simulink model "A_Novel_Converter_Topology_for_Stand_Alone"  (Simulink 7.3)
settings: Solver=ode45  StartTime=0.0  StopTime=0.7  MaxStep=1e-6  RelTol=1e-3
libraries: powerlib x20
settings Model: Creator=KARTHIK  LastModifiedBy=91889
settings DebuggingCC: FcnCallInpInsideContextMsg=Enable All  StrictBusMsg=ErrorLevel1
settings GRTTargetCC: CombineOutputUpdateFcns=on

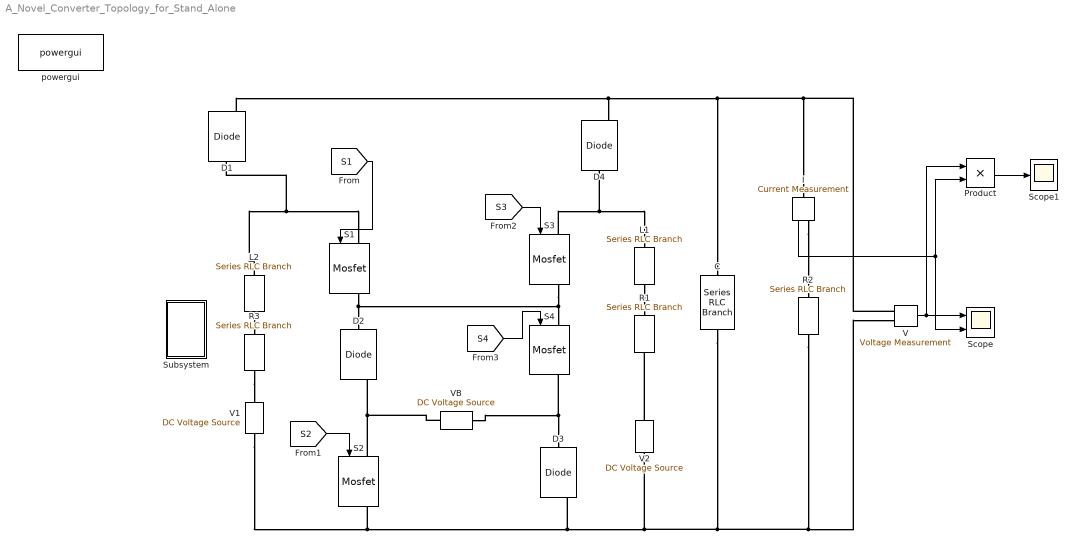
== system A_Novel_Converter_Topology_for_Stand_Alone ==
  C : powerlib/Elements/Series RLC Branch  DialogController=POWERSYS.PowerSysDialog  PhysicalDomain=powersysdomain  SubClassName=unknown  LeftPortType=p1  RightPortType=p1  LConnTagsString=__new0  RConnTagsString=__new0  BranchType=C  Resistance=1  Inductance=1e-3  SetiL0=off  InitialCurrent=0  Capacitance=200e-6  Setx0=off  InitialVoltage=0  Measurements=None
  D{1..4} (4 alike) : powerlib/Power Electronics/Diode  DialogController=POWERSYS.PowerSysDialog  SystemSampleTime=-1  Ron=0.001  Lon=0  Vf=0.8  IC=0  UseSnubber=off  Rs=500  Cs=250e-9  Measurements=on
  I : powerlib/Measurements/Current Measurement  DialogController=POWERSYS.PowerSysDialog  SystemSampleTime=-1  PhasorSimulation=off  OutputType=Complex  PSBequivalent=0
  L1 : powerlib/Elements/Series RLC Branch  DialogController=POWERSYS.PowerSysDialog  PhysicalDomain=powersysdomain  SubClassName=unknown  LeftPortType=p1  RightPortType=p1  LConnTagsString=__new0  RConnTagsString=__new0  BranchType=L  Resistance=1  Inductance=6e-3  SetiL0=off  InitialCurrent=0  Capacitance=1e-6  Setx0=off  InitialVoltage=0  Measurements=None
  L2 : powerlib/Elements/Series RLC Branch  DialogController=POWERSYS.PowerSysDialog  PhysicalDomain=powersysdomain  SubClassName=unknown  LeftPortType=p1  RightPortType=p1  LConnTagsString=__new0  RConnTagsString=__new0  BranchType=L  Resistance=1  Inductance=6e-3  SetiL0=off  InitialCurrent=0  Capacitance=1e-6  Setx0=off  InitialVoltage=0  Measurements=None
  Product : Product  RndMeth=Zero
  R1 : powerlib/Elements/Series RLC Branch  DialogController=POWERSYS.PowerSysDialog  PhysicalDomain=powersysdomain  SubClassName=unknown  LeftPortType=p1  RightPortType=p1  LConnTagsString=__new0  RConnTagsString=__new0  BranchType=R  Resistance=0.4  Inductance=1e-3  SetiL0=off  InitialCurrent=0  Capacitance=1e-6  Setx0=off  InitialVoltage=0  Measurements=None
  R2 : powerlib/Elements/Series RLC Branch  DialogController=POWERSYS.PowerSysDialog  PhysicalDomain=powersysdomain  SubClassName=unknown  LeftPortType=p1  RightPortType=p1  LConnTagsString=__new0  RConnTagsString=__new0  BranchType=R  Resistance=50  Inductance=1e-3  SetiL0=off  InitialCurrent=0  Capacitance=1e-6  Setx0=off  InitialVoltage=0  Measurements=None
  R3 : powerlib/Elements/Series RLC Branch  DialogController=POWERSYS.PowerSysDialog  PhysicalDomain=powersysdomain  SubClassName=unknown  LeftPortType=p1  RightPortType=p1  LConnTagsString=__new0  RConnTagsString=__new0  BranchType=R  Resistance=0.4  Inductance=1e-3  SetiL0=off  InitialCurrent=0  Capacitance=1e-6  Setx0=off  InitialVoltage=0  Measurements=None
  S{1..4} (4 alike) : powerlib/Power Electronics/Mosfet  DialogController=POWERSYS.PowerSysDialog  SystemSampleTime=-1  Ron=0.1  Lon=0  Rd=0.01  Vfd=0  IC=0  Rs=1e5  Cs=inf  Measurements=on
  Scope : Scope  NumInputPorts=2
      settings: YMin=297.5~-5  YMax=305~5
  Scope1 : Scope
      settings: YMin=594  YMax=608
  Subsystem : Subsystem
  V : powerlib/Measurements/Voltage Measurement  DialogController=POWERSYS.PowerSysDialog  SystemSampleTime=-1  PhasorSimulation=off  OutputType=Complex  PSBequivalent=0
  V1 : powerlib/Electrical Sources/DC Voltage Source  DialogController=POWERSYS.PowerSysDialog  SystemSampleTime=-1  Amplitude=100  Measurements=Voltage
  V2 : powerlib/Electrical Sources/DC Voltage Source  DialogController=POWERSYS.PowerSysDialog  SystemSampleTime=-1  Amplitude=100  Measurements=Voltage
  VB : powerlib/Electrical Sources/DC Voltage Source  DialogController=POWERSYS.PowerSysDialog  SystemSampleTime=-1  Amplitude=82  Measurements=None
  powergui : powerlib/powergui  Priority=1  SystemSampleTime=-1  SimulationMode=Discrete  SampleTime=1e-6  frequency=60  SPID=off  DisableSnubberDevices=off  DisableRonSwitches=off  DisableVfSwitches=off  SwTol=0  Interpol=off  frequencyindice=0  echomessages=off  HookPort=off  DisplayEquations=off  FunctionMessages=off  EnableUseOfTLC=off  x0status=blocks  RestoreLinks=warning  Frange=[0:2:500]  Ylog=off  Xlog=on  ShowGrid=off  save=off  variable=ZData  ZoomFFT=off  StartTime=0.0  cycles=1  DisplayStyle=1  fundamental=60  FreqAxis=off  MaxFrequency=1000  frequencyindicesteady=1  RmsSteady=1  display=off  Ts=0  methode=off
  wires:
  V/1 -> Scope/1, Product/1
  I/1 -> Scope/2, Product/2
  [S1] -> S1/1
  [S2] -> S2/1
  [S3] -> S3/1
  [S4] -> S4/1
  Product/1 -> Scope1/1
  connections:
  R3/RConn1 -- V1/RConn1
  L2/RConn1 -- R3/LConn1
  S1/LConn1 -- L2/LConn1 -- D1/LConn1
  S1/RConn1 -- D2/LConn1 -- S3/RConn1 -- S4/LConn1
  S2/LConn1 -- D2/RConn1 -- VB/RConn1
  R2/RConn1 -- C/RConn1 -- V1/LConn1 -- S2/RConn1 -- D3/RConn1 -- V2/LConn1 -- V/LConn2
  VB/LConn1 -- S4/RConn1 -- D3/LConn1
  L1/RConn1 -- R1/LConn1
  V2/RConn1 -- R1/RConn1
  S3/LConn1 -- L1/LConn1 -- D4/LConn1
  V/LConn1 -- D1/RConn1 -- D4/RConn1 -- C/LConn1 -- I/LConn1
  I/RConn1 -- R2/LConn1

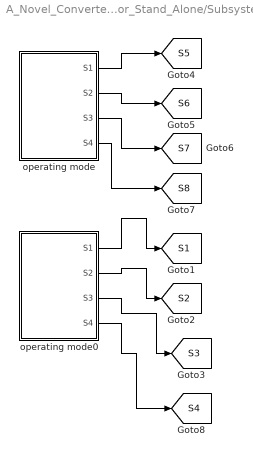
== system A_Novel_Converter_Topology_for_Stand_Alone/Subsystem ==
  operating mode : Subsystem
  operating mode0 : Subsystem
  tag scope: S1=global, S2=global, S3=global, S4=global, S5=global, S6=global, S7=global, S8=global
  wires:
  operating mode0/1(S1) -> [S1]
  operating mode0/2(S2) -> [S2]
  operating mode0/4(S4) -> [S4]
  operating mode/1(S1) -> [S5]
  operating mode/2(S2) -> [S6]
  operating mode/3(S3) -> [S7]
  operating mode/4(S4) -> [S8]
  operating mode0/3(S3) -> [S3]

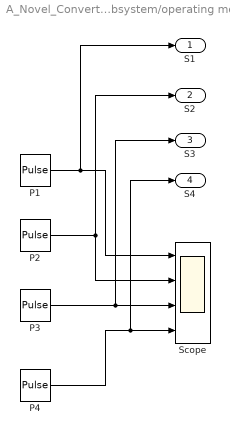
== system A_Novel_Converter_Topology_for_Stand_Alone/Subsystem/operating mode ==
  P1 : DiscretePulseGenerator  PulseType=Time based  Amplitude=1  Period=5e-5  PulseWidth=50  PhaseDelay=0  SampleTime=1
  P2 : DiscretePulseGenerator  PulseType=Time based  Amplitude=1  Period=5e-5  PulseWidth=75  PhaseDelay=0  SampleTime=1
  P3 : DiscretePulseGenerator  PulseType=Time based  Amplitude=1  Period=5e-5  PulseWidth=75  PhaseDelay=0  SampleTime=1
  P4 : DiscretePulseGenerator  PulseType=Time based  Amplitude=1  Period=5e-5  PulseWidth=25  PhaseDelay=0  SampleTime=1
  Scope : Scope  NumInputPorts=4
      settings: YMin=-5~-5~-5~-5  YMax=5~5~5~5
  S1 : Outport
  S2 : Outport  Port=2
  S3 : Outport  Port=3
  S4 : Outport  Port=4
  wires:
  P1/1 -> Scope/1, S1/1
  P2/1 -> Scope/2, S2/1
  P3/1 -> Scope/3, S3/1
  P4/1 -> Scope/4, S4/1

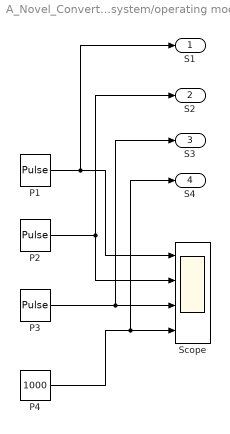
== system A_Novel_Converter_Topology_for_Stand_Alone/Subsystem/operating mode0 ==
  P1 : DiscretePulseGenerator  PulseType=Time based  Amplitude=1  Period=5e-5  PulseWidth=50  PhaseDelay=0  SampleTime=1
  P2 : DiscretePulseGenerator  PulseType=Time based  Amplitude=1  Period=5e-5  PulseWidth=75  PhaseDelay=0  SampleTime=1
  P3 : DiscretePulseGenerator  PulseType=Time based  Amplitude=1  Period=5e-5  PulseWidth=25  PhaseDelay=0  SampleTime=1
  P4 : Constant  Value=1000  VectorParams1D=off
  Scope : Scope  NumInputPorts=4
      settings: YMin=-5~-5~-5~-5  YMax=5~5~5~5
  S1 : Outport
  S2 : Outport  Port=2
  S3 : Outport  Port=3
  S4 : Outport  Port=4
  wires:
  P1/1 -> Scope/1, S1/1
  P2/1 -> Scope/2, S2/1
  P3/1 -> Scope/3, S3/1
  P4/1 -> Scope/4, S4/1
